simulink model "DC_Motor_block"  (R2020a)
settings: Solver=VariableStepAuto  StartTime=0.0  StopTime=10.0  RelTol=1e-3
values from neighbouring files (symbols this model uses):
  b = 0.1    [open_loop.m]    (also in pid_controller.m; system_eq.m)
  J = 0.01    [open_loop.m]    (also in pid_controller.m; system_eq.m)
  K = 0.01    [open_loop.m]    (also in pid_controller.m; system_eq.m)
  L = 0.5    [open_loop.m]    (also in pid_controller.m; system_eq.m)
  R = 1    [open_loop.m]    (also in pid_controller.m; system_eq.m)
settings Model: Creator=Maria  LastModifiedBy=Maria

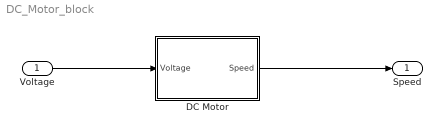
== system DC_Motor_block ==
  Voltage : Inport
  DC Motor : Subsystem
  Speed : Outport
  wires:
  Voltage/1 -> DC Motor/1(Voltage)
  DC Motor/1(Speed) -> Speed/1

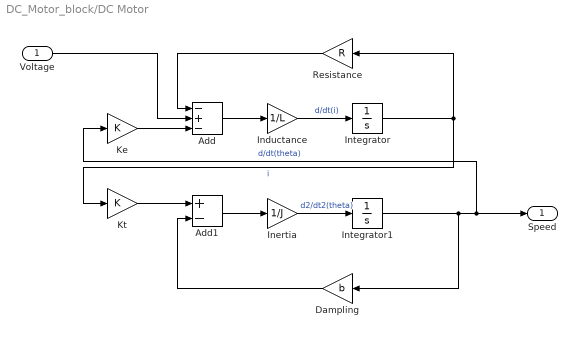
== system DC_Motor_block/DC Motor ==
  Voltage : Inport
  Add : Sum  Inputs=-+-
  Add1 : Sum  Inputs=+-
  Dampling : Gain  Gain=b
  Inductance : Gain  Gain=1/L
  Inertia : Gain  Gain=1/J
  Integrator : Integrator
  Integrator1 : Integrator
  Ke : Gain  Gain=K
  Kt : Gain  Gain=K
  Resistance : Gain  Gain=R
  Speed : Outport
  wires:
  Inductance/1 -> Integrator/1  "d/dt(i)"
  Add/1 -> Inductance/1
  Ke/1 -> Add/3
  Inertia/1 -> Integrator1/1  "d2/dt2(theta)"
  Add1/1 -> Inertia/1
  Voltage/1 -> Add/2
  Integrator/1 -> Resistance/1, Kt/1  "i"
  Integrator1/1 -> Speed/1, Ke/1, Dampling/1  "d/dt(theta)"
  Resistance/1 -> Add/1
  Kt/1 -> Add1/1
  Dampling/1 -> Add1/2
